simulink model "EKF_Sim_FAEKF"  (R2018a)
settings: Solver=ode4  StartTime=time_start  StopTime=time_end  FixedStep=time_step  MaxStep=0.1  RelTol=1e-6  AbsTol=1e-6
values from neighbouring files (symbols this model uses):
  FUZZY_props =     [FAEKF_FuzzyProps.mat]    (also in FFNAV_FAEKF_RunSim.m = FFNAV_FAEKF_FuzzyInitialize(MSFplot_flag))
  GPS_r_STD = 10*GPS_r_STD    [FFNAV_FAEKF_RunSim.m]
  GPS_v_STD = 10*GPS_v_STD    [FFNAV_FAEKF_RunSim.m]
  N_window = 30    [FFNAV_FAEKF_RunSim.m]
  Q0 = 10*Q0    [FFNAV_FAEKF_RunSim.m]
  Q_adapt = Q0    [FFNAV_FAEKF_FuzzyAdapt.m]    (also in FFNAV_FAEKF_RunSim.m = 0)
  R0 = R0    [FFNAV_FAEKF_RunSim.m]
  R_adapt = R0*beta^(-2*(k))    [FFNAV_FAEKF_FuzzyAdapt.m]    (also in FFNAV_FAEKF_RunSim.m = 0)
  time_step = 1    [FFNAV_FAEKF_RunSim.m]
undefined symbols (not defined in the file or in its folder): COE_chaser, COE_target, Constants, mu, n, PropOptions_chaser, PropOptions_target, theta0_target
libraries: dspindex x9, dspstat3 x7, dspmtrx3 x1
(part 2 of 2)

== matlab function EKF_Sim_FAEKF/Kalman Filter/EKF/EKF Correction/MATLAB Function ==
  data: sensors input; state_priori input; output output; R input
 function output = USE_FAEKF_Correction(sensors, state_priori, R)
%% USE_EKF ===============================================================
% ========================================================================
% Description: This function calls the FFNAV_EKF Function, which completes 
% the covariance propagation and correction phases of the EKF algorithm. 
% The output is then passed back to the simulink model.

output = zeros(243,1);
[output] = FFNAV_FAEKF_Correction(state_priori, sensors, R);
end
% ========================================================================

== matlab function EKF_Sim_FAEKF/Kalman Filter/EKF/EKF Propagation/MATLAB Function ==
  data: state_pre input; output output; Q input; time_step parameter; mu parameter
 function output  = USE_FAEKF_Propagation(state_pre, Q, time_step, mu)
%% USE_EKF ===============================================================
% ========================================================================
% Description: This function calls the FFNAV_EKF Function, which completes 
% the covariance propagation and correction phases of the EKF algorithm. 
% The output is then passed back to the simulink model.

output = zeros(110,1);
output = FFNAV_FAEKF_Propagation(state_pre, time_step, mu, Q);
end
% ========================================================================

== matlab function EKF_Sim_FAEKF/Kalman Filter/MLE-EKF/MATLAB Function ==
  data: Storage_out output; Storage_in input; state_pre input; sensors input; EKF_out output; Q input; R input; L output; Q_update output; R_update output; time_step parameter; mu parameter; Q_adapt parameter; R_adapt parameter
  function [Storage_out, EKF_out, L, Q_update, R_update] = ...
      USE_EKF_MLE(Storage_in,state_pre,sensors,Q,R,time_step,mu,Q_adapt,R_adapt)
%% USE_EKF ===============================================================
% Description: This function calls the FFNAV_EKF Function, which completes 
% the covariance propagation and correction phases of the EKF algorithm. 
% The output is then passed back to the simulink model.

EKF_out     = zeros(243,1);
Storage_out = zeros(334,1);
Q_update    = zeros(10,10);
R_update    = zeros(7,7);

[EKF_out, Storage_out, L, Q_update, R_update] = ...
    FFNAV_EKF_MLE(Storage_in,time_step,mu,state_pre,sensors,Q,R,Q_adapt,R_adapt);
end
% ========================================================================

== matlab function EKF_Sim_FAEKF/Kalman Filter/FAEKF/Adaptations/Theoretical Covariances ==
  data: Pr_vector input; y output
function y = fcn(Pr_vector)
%#codegen

Pr_theo = [         Pr_vector(1:7)'
                    Pr_vector(8:14)'
                    Pr_vector(15:21)'
                    Pr_vector(22:28)'
                    Pr_vector(29:35)'
                    Pr_vector(36:42)'
                    Pr_vector(43:49)'];
                
Pr_theo_diag = diag(Pr_theo);
   
y = Pr_theo_diag;

== matlab function EKF_Sim_FAEKF/Kalman Filter/FAEKF/Adaptations/USE_FuzzyAdapt ==
  data: state_pre input; Pr_theo input; Pr_smooth input; residuals input; time input; FUZZY_props parameter; Q_pre input; R_pre input; time_step parameter; mu parameter; Q0 parameter; R0 parameter; NIS output; deltaDOD output; DOD_true output; Q output; R output; epsilon_Q output; epsilon_R output; R_adapt parameter; Q_adapt parameter
   function [NIS, deltaDOD, DOD_true, Q,R, epsilon_Q, epsilon_R] = ...
       USE_FuzzyAdapt(state_pre, Pr_theo, Pr_smooth, residuals, ...
     time, FUZZY_props, Q_pre, R_pre, time_step, mu, Q0, R0, R_adapt, Q_adapt)
%% USE_EKF ===============================================================
% ========================================================================
% Description: This block calls the FFNAV_EKF Fuzzy Adaptation function, 
% which calculates an update of the process and measurement noise  
% covariance matrices.

Q = zeros(10,10);
R = zeros(7,7);

[Q, R, NIS, deltaDOD, DOD_true, epsilon_Q, epsilon_R] = ...
    FFNAV_FAEKF_FuzzyAdapt(state_pre, Pr_theo, Pr_smooth, residuals, ...
    time_step, mu, Q0, R0, Q_pre, R_pre, time, FUZZY_props, Q_adapt, R_adapt);

end
% ========================================================================

== matlab function EKF_Sim_FAEKF/Kalman Filter/FAEKF/EKF Correction/MATLAB Function ==
  data: sensors input; input_priori input; output output; R input
 function output = USE_FAEKF_Correction(sensors, input_priori, R)
%% USE_EKF ===============================================================
% ========================================================================
% Description: This function calls the FFNAV_EKF Function, which completes 
% the covariance propagation and correction phases of the EKF algorithm. 
% The output is then passed back to the simulink model.

output = zeros(243,1);
[output] = FFNAV_FAEKF_Correction(input_priori, sensors, R);
end
% ========================================================================

== matlab function EKF_Sim_FAEKF/Kalman Filter/FAEKF/EKF Propagation/MATLAB Function ==
  data: state_pre input; output output; Q input; time_step parameter; mu parameter
 function output = USE_FAEKF_Propagation(state_pre, Q, time_step, mu)
%% USE_EKF ===============================================================
% ========================================================================
% Description: This function calls the FFNAV_EKF Function, which completes 
% the covariance propagation and correction phases of the EKF algorithm. 
% The output is then passed back to the simulink model.

output = zeros(110,1);
output = FFNAV_FAEKF_Propagation(state_pre, time_step, mu, Q);
end
% ========================================================================
